simulink model "model"  (R2025a)
settings: Solver=VariableStepAuto  StartTime=0.0  StopTime=13  RelTol=1e-3
InitFcn:
  | r=0.315
  | m_c=1477
  | m_v=1645
  | n_g=9.73
  | eta_g=0.98
  | A=133.3
  | B=0.7094
  | C=0.491
  | 
  | v_rated=43.61
  | P_rated=80e3
  | T_rated=254
  | 
  | theta=0
  | v_air=0
  | m_i = m_c*(0.04 + 0.0025*n_g^2)
  | m=m_v+m_i
libraries: simulink_extras x1
settings Model: Creator=jw  LastModifiedBy=jackh
settings SolverCC: AlgebraicLoopSolver=TrustRegion
settings DataIOCC: ReturnWorkspaceOutputs=off
settings DebuggingCC: UnconnectedInputMsg=warning  UnconnectedOutputMsg=warning  UnconnectedLineMsg=warning  ArithmeticOperatorsInVariantConditions=warning
settings ModelReferenceCC: EnableRefExpFcnMdlSchedulingChecks=on
settings SFSimCC: SimUseLocalCustomCode=off  CustomCodeUndefinedFunction=UseInterfaceOnly
settings RTWCC: RTWUseLocalCustomCode=off  GPUComputeCapability=3.5

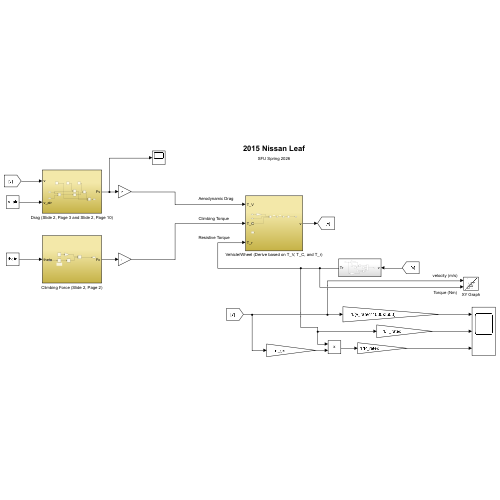
[thumbnail: Simulink's stored preview of the top-level diagram]
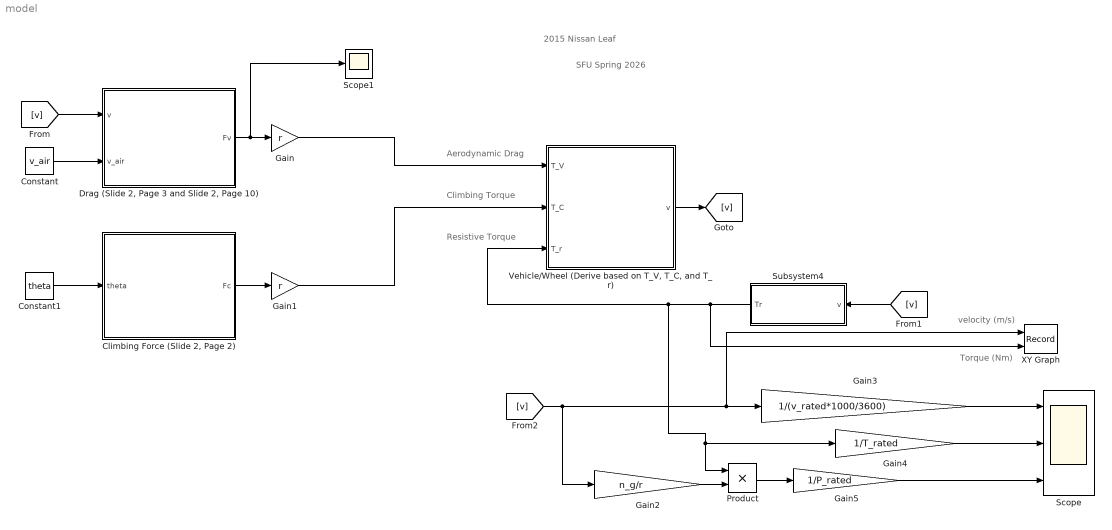
== system model ==
  note: Torque (Nm)
  note: velocity (m/s)
  note: Aerodynamic Drag
  note: Climbing Torque
  note: Resistive Torque
  note: 2015 Nissan Leaf
  note: SFU Spring 2026
  "Climbing Force (Slide 2, Page 2)" : Subsystem
  Constant : Constant  Value=v_air
  Constant1 : Constant  Value=theta
  "Drag (Slide 2, Page 3 and Slide 2, Page 10)" : Subsystem
  Gain : Gain  Gain=r
  Gain1 : Gain  Gain=r
  Gain2 : Gain  Gain=n_g/r
  Gain3 : Gain  Gain=1/(v_rated*1000/3600)
  Gain4 : Gain  Gain=1/T_rated
  Gain5 : Gain  Gain=1/P_rated
  Product : Product
  Scope : Scope  NumInputPorts=3
      settings: ActiveDisplayYMinimum=-0.30089419778032517  ActiveDisplayYMaximum=2.7080477800229268
  Scope1 : Scope
      settings: ActiveDisplayYMinimum=-1  ActiveDisplayYMaximum=1
  Subsystem4 : Subsystem
  "Vehicle/Wheel (Derive based on T_V, T_C, and T_r)" : Subsystem
  XY Graph : Record  NumPorts=2.0  FileSettingsInternal="{\"entries\":[{\"content\":{\"excelSettings\":{\"content\":{},\"type\":\"Streamout.ExcelSettings\"},\"parquetSettings\":{\"content\":{},\"type\":\"Streamout.ParquetSettings\"}},\"type\":\"Streamout.FileSettingStorage\",\"uuid\":\"\"}],\"packageUris\":[\"http:\\/\\/schema.mathworks.com\\/mf0\\/streamout_blocks\\/R2020a\"],\"version\":\"1.0\"}"  FrameSettings=[0, 0]  Layout=[1 1]  SignalsInternal="{\"entries\":[{\"content\":{\"signals\":[{\"content\":{\"blockPath\":[],\"dimensions\":[1],\"domain\":\"\",\"lineColor\":\"#a2142f\",\"plots\":[ 1 ],\"port\":1,\"signalID\":1,\"signalName\":\"From2\"},\"type\":\"RecordBlkView.Signal\",\"uuid\":\"\"},{\"content\":{\"blockPath\":[],\"dimensions\":[1],\"domain\":\"\",\"lineColor\":\"#139fff\",\"plots\":[ 1 ],\"port\":2,\"signalID\":2,\"signalName\":\"Subsystem4\"},\"type\":\"RecordBlkView.Signal\",\"uuid\":\"\"}]},\"type\":\"RecordBlkView.InputSignals\",\"uuid\":\"\"}],\"packageUris\":[\"http:\\/\\/schema.mathworks.com\\/mf0\\/streamout_blocks\\/R2020a\"],\"version\":\"1.0\"}"  VisualizationBindings="{\"xyplotplugin\":{\"info\":[{\"series\":[{\"bindingParametersList\":[{\"parameter\":\"X-Axis\",\"signalID\":1,\"signalName\":\"From2\"},{\"parameter\":\"Y-Axis\",\"signalID\":2,\"signalName\":\"Subsystem4\"}],\"seriesID\":0}],\"subplotID\":1}]}}"  CompatibilityTag=XY
  wires:
  "Drag (Slide 2, Page 3 and Slide 2, Page 10)"/1(Fv) -> Scope1/1, Gain/1
  "Climbing Force (Slide 2, Page 2)"/1(Fc) -> Gain1/1
  "Vehicle/Wheel (Derive based on T_V, T_C, and T_r)"/1(v) -> [v]
  [v] -> "Drag (Slide 2, Page 3 and Slide 2, Page 10)"/1(v)
  Constant/1 -> "Drag (Slide 2, Page 3 and Slide 2, Page 10)"/2(v_air)
  Constant1/1 -> "Climbing Force (Slide 2, Page 2)"/1(theta)
  Gain/1 -> "Vehicle/Wheel (Derive based on T_V, T_C, and T_r)"/1(T_V)
  Gain1/1 -> "Vehicle/Wheel (Derive based on T_V, T_C, and T_r)"/2(T_C)
  Subsystem4/1(Tr) -> XY Graph/2, Product/1, Gain4/1, "Vehicle/Wheel (Derive based on T_V, T_C, and T_r)"/3(T_r)
  [v] -> XY Graph/1, Gain3/1, Gain2/1
  Gain2/1 -> Product/2
  Gain4/1 -> Scope/2
  Product/1 -> Gain5/1
  Gain5/1 -> Scope/3
  Gain3/1 -> Scope/1
  [v] -> Subsystem4/1(v)

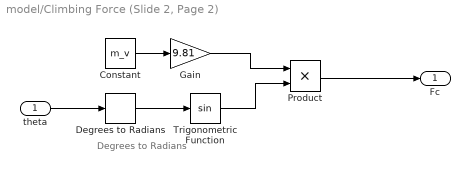
== system model/Climbing Force (Slide 2, Page 2) ==
  note: Degrees to
      | Radians
  theta : Inport
  Constant : Constant  Value=m_v
  Degrees to Radians : simulink_extras/Transformations/Degrees to Radians
  Gain : Gain  Gain=9.81
  Product : Product
  Trigonometric Function : Trigonometry
  Fc : Outport  VectorParamsAs1DForOutWhenUnconnected=off
  wires:
  Trigonometric Function/1 -> Product/2
  Constant/1 -> Gain/1
  Gain/1 -> Product/1
  theta/1 -> Degrees to Radians/1
  Degrees to Radians/1 -> Trigonometric Function/1
  Product/1 -> Fc/1

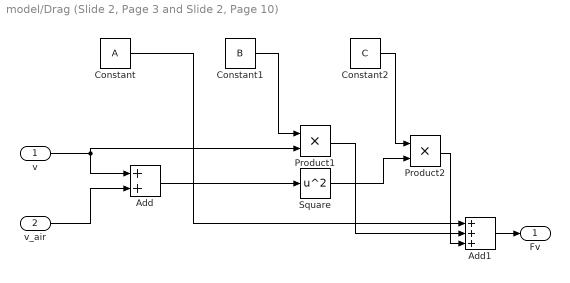
== system model/Drag (Slide 2, Page 3 and Slide 2, Page 10) ==
  v : Inport
  v_air : Inport  Port=2
  Add : Sum
  Add1 : Sum  Inputs=+++
  Constant : Constant  Value=A
  Constant1 : Constant  Value=B
  Constant2 : Constant  Value=C
  Product1 : Product
  Product2 : Product
  Square : Math  Operator=square
  Fv : Outport  VectorParamsAs1DForOutWhenUnconnected=off
  wires:
  v/1 -> Add/1, Product1/2
  v_air/1 -> Add/2
  Add1/1 -> Fv/1
  Add/1 -> Square/1
  Constant1/1 -> Product1/1
  Constant2/1 -> Product2/1
  Product1/1 -> Add1/2
  Product2/1 -> Add1/3
  Constant/1 -> Add1/1
  Square/1 -> Product2/2

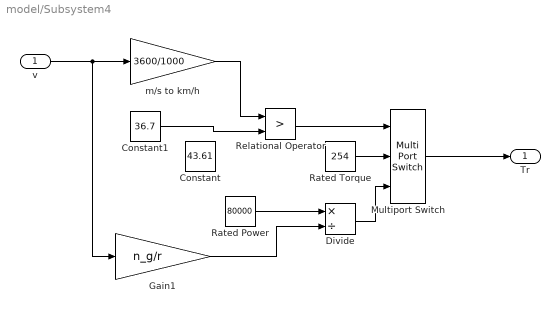
== system model/Subsystem4 ==
  v : Inport
  Constant : Constant  Value=43.61
  Constant1 : Constant  Value=36.7
  Divide : Product  Inputs=*/
  Gain1 : Gain  Gain=n_g/r
  Multiport Switch : MultiPortSwitch  DataPortOrder=Zero-based contiguous  Inputs=2  zeroidx=on  SaturateOnIntegerOverflow=off  InputSameDT=off
  Rated Power : Constant  Value=80000
  Rated Torque : Constant  Value=254
  Relational Operator : RelationalOperator  Operator=>  OutDataTypeStr=boolean  RndMeth=Simplest  InputSameDT=off
  m/s to km/h : Gain  Gain=3600/1000
  Tr : Outport  VectorParamsAs1DForOutWhenUnconnected=off
  wires:
  Multiport Switch/1 -> Tr/1
  m/s to km/h/1 -> Relational Operator/1
  Rated Torque/1 -> Multiport Switch/2
  Relational Operator/1 -> Multiport Switch/1
  Rated Power/1 -> Divide/1
  v/1 -> Gain1/1, m/s to km/h/1
  Divide/1 -> Multiport Switch/3
  Gain1/1 -> Divide/2
  Constant1/1 -> Relational Operator/2

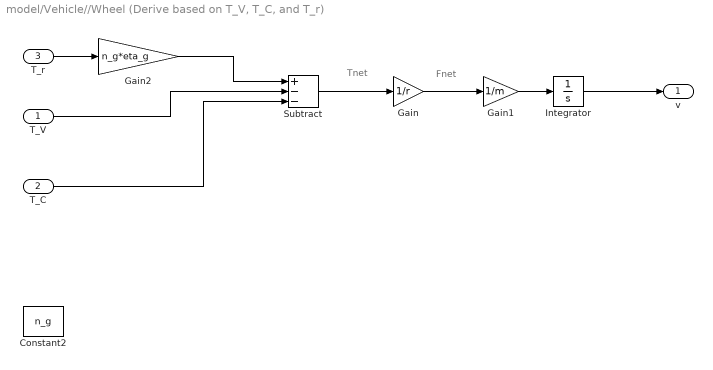
== system model/Vehicle//Wheel (Derive based on T_V, T_C, and T_r) ==
  note: Fnet
  note: Tnet
  T_V : Inport
  T_C : Inport  Port=2
  T_r : Inport  Port=3
  Constant2 : Constant  Value=n_g
  Gain : Gain  Gain=1/r
  Gain1 : Gain  Gain=1/m
  Gain2 : Gain  Gain=n_g*eta_g
  Integrator : Integrator
  Subtract : Sum  Inputs=+--
  v : Outport  VectorParamsAs1DForOutWhenUnconnected=off
  wires:
  T_r/1 -> Gain2/1
  Gain2/1 -> Subtract/1
  T_V/1 -> Subtract/2
  T_C/1 -> Subtract/3
  Subtract/1 -> Gain/1
  Gain/1 -> Gain1/1
  Gain1/1 -> Integrator/1
  Integrator/1 -> v/1
